simulink model "Gradient_Descent_Sleep_Line_Search"  (R2015a)
settings: Solver=ode3  StartTime=0.0  StopTime=350  FixedStep=0.01  MaxStep=0.01  RelTol=1e-3
values from neighbouring files (symbols this model uses):
  H0 = interp1q(Periodic_Solution(:,1),Periodic_Solution(:,4),time_shift(n))    [Gradient_Descent_Controllable_Sleeping.m]
  Periodic_Solution = Periodic_Solution(Initial_Time*100+1:end,:)    [Gradient_Descent_Controllable_Sleeping.m]    (also in Periodic_Solution_JFK_u_1000lux.mat = [0 0.00999999999999 0.02 0.03 0.04 0.05 0.0599999999999 0.06)
  Sleep0 = 0    [Gradient_Descent_Controllable_Sleeping.m]
  Sleep_update = Sleep    [Gradient_Descent_Controllable_Sleeping.m]
  tol = 0.01    [Gradient_Descent_Controllable_Sleeping.m]
  u_update = u    [Gradient_Descent_Controllable_Sleeping.m]
  x0 = interp1q(Periodic_Solution(:,1),Periodic_Solution(:,2),time_shift(n))    [Gradient_Descent_Controllable_Sleeping.m]
  xc0 = interp1q(Periodic_Solution(:,1),Periodic_Solution(:,3),time_shift(n))    [Gradient_Descent_Controllable_Sleeping.m]
settings Model: Creator=wangf7  LastModifiedBy=Jiawei Yin
settings OptimizationCC: ExpressionDepthLimit=2147483647
settings DebuggingCC: AlgebraicLoopMsg=none  ArtificialAlgebraicLoopMsg=none  UnderspecifiedInitializationDetection=Classic  MergeDetectMultiDrivingBlocksExec=none  SolverPrmCheckMsg=warning  StateNameClashWarn=warning

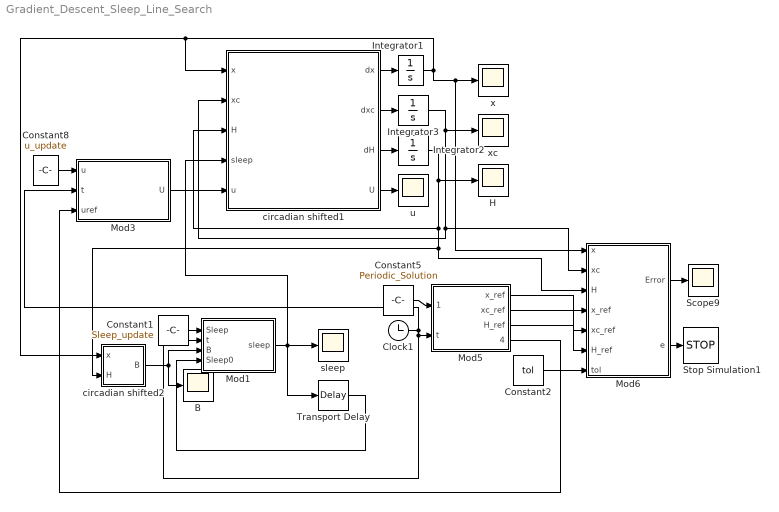
== system Gradient_Descent_Sleep_Line_Search ==
  B : Scope
      settings: TimeRange=auto  MaxDataPoints=5000000000  SaveName=B_plus  YMin=0.1808  YMax=0.82676  SampleTime=-1  DataFormat=Array
  Clock1 : Clock
  Constant1 : Constant  Value=Sleep_update
  Constant2 : Constant  Value=tol
  Constant5 : Constant  Value=Periodic_Solution
  Constant8 : Constant  Value=u_update
  H : Scope
      settings: TimeRange=auto  MaxDataPoints=5000000000  SaveName=H_plus  YMin=0.55428  YMax=0.67222  SampleTime=-1  DataFormat=Array
  Integrator1 : Integrator  InitialCondition=x0
  Integrator2 : Integrator  InitialCondition=H0
  Integrator3 : Integrator  InitialCondition=xc0
  Mod1 : MATLAB Function  TreatAsAtomicUnit=on
      settings: PermitHierarchicalResolution=ParametersOnly
  Mod3 : MATLAB Function  TreatAsAtomicUnit=on
      settings: PermitHierarchicalResolution=ParametersOnly
  Mod5 : MATLAB Function  TreatAsAtomicUnit=on
      settings: PermitHierarchicalResolution=ParametersOnly
  Mod6 : MATLAB Function  TreatAsAtomicUnit=on
      settings: PermitHierarchicalResolution=ParametersOnly
  Scope9 : Scope
      settings: TimeRange=auto  MaxDataPoints=5000000000  SaveName=Error_plus  YMin=-0.4029  YMax=6.32555  SampleTime=-1  DataFormat=Array
  Stop Simulation1 : Stop
  Transport Delay : TransportDelay  DelayTime=.01  InitialOutput=Sleep0
  circadian shifted1 : MATLAB Function  TreatAsAtomicUnit=on
      settings: PermitHierarchicalResolution=ParametersOnly
  circadian shifted2 : MATLAB Function  TreatAsAtomicUnit=on
      settings: PermitHierarchicalResolution=ParametersOnly
  sleep : Scope
      settings: TimeRange=auto  MaxDataPoints=5000000000  SaveName=sleep_plus  YMin=-0.125  YMax=1.125  SampleTime=-1  DataFormat=Array
  u : Scope
      settings: TimeRange=auto  MaxDataPoints=5000000000  SaveName=u_plus  YMin=0.55428  YMax=0.67222  SampleTime=-1  DataFormat=Array
  x : Scope
      settings: TimeRange=auto  MaxDataPoints=5000000000  SaveName=x_plus  YMin=-1.43661  YMax=1.34945  SampleTime=-1  DataFormat=Array
  xc : Scope
      settings: TimeRange=auto  MaxDataPoints=5000000000  SaveName=xc_plus  YMin=0.55428  YMax=0.67222  SampleTime=-1  DataFormat=Array
  wires:
  circadian shifted1/1(dx) -> Integrator1/1
  circadian shifted1/2(dxc) -> Integrator3/1
  Integrator1/1 -> x/1, Mod6/1(x), circadian shifted1/1(x), circadian shifted2/1(x)
  Integrator3/1 -> circadian shifted1/2(xc), Mod6/2(xc), xc/1
  Constant5/1 -> Mod5/1(Periodic_Solution)
  Mod6/2(e) -> Stop Simulation1/1
  Mod6/1(Error) -> Scope9/1
  Mod5/3(H_ref) -> Mod6/6(H_ref)
  Constant2/1 -> Mod6/7(tol)
  Constant1/1 -> Mod1/1(Sleep)
  Clock1/1 -> Mod1/2(t), Mod5/2(t), Mod3/2(t)
  Mod1/1(sleep) -> circadian shifted1/4(sleep), Transport Delay/1, sleep/1
  circadian shifted2/1(B) -> Mod1/3(B), B/1
  Transport Delay/1 -> Mod1/4(Sleep0)
  circadian shifted1/3(dH) -> Integrator2/1
  Integrator2/1 -> Mod6/3(H), circadian shifted2/2(H), circadian shifted1/3(H), H/1
  Mod5/1(x_ref) -> Mod6/4(x_ref)
  Mod5/2(xc_ref) -> Mod6/5(xc_ref)
  Constant8/1 -> Mod3/1(u)
  Mod3/1(U) -> circadian shifted1/5(u)
  circadian shifted1/4(U) -> u/1
  Mod5/4(Sleep_ref) -> Mod3/3(uref)

== matlab function Gradient_Descent_Sleep_Line_Search/circadian shifted1 ==
  data: x input; xc input; H input; sleep input; u input; dx output; dxc output; dH output; U output
function [ dx,dxc,dH,U] = fcn(x,xc,H,sleep,u)
%#eml

tr=18.2;
td=4.2;

q = 1/3;
taux = 24.2;
k = 0.55;
mu=0.13;
U=u*(1-sleep);
B = u*(1-0.4*x)*(1-0.4*xc)*(1-sleep);

dx = (pi/12)*(xc + B  + mu*(1/3*x + 4/3*x^3 - 256/105*x^7));
dxc = (pi/12)*(q*B *xc - (24/(taux*0.99729))^2*x - k*B*x);
dH = (1-sleep)*(1-H)/tr-(H*sleep)/td;

== matlab function Gradient_Descent_Sleep_Line_Search/Mod1 ==
  data: Sleep input; sleep output; t input; B input; Sleep0 input
function sleep = fcn(Sleep,t,B,Sleep0)
%#codegen
if t<=Sleep(end,1)
    sleep=interp1q(Sleep(:,1),Sleep(:,2),t);
    if sleep==0 && Sleep0==1
        if B>0.27
            sleep=1;
        end
    elseif sleep==1 && Sleep0==0
        if B<0.67
            sleep=0;
        end
    end
    if B>0.77
        sleep=1;
    elseif B<0.17
        sleep=0;
    end
else
    sleep=Sleep0;
    if B>0.67
        sleep=1;
    elseif B<0.17
        sleep=0;
    end
end

== matlab function Gradient_Descent_Sleep_Line_Search/circadian shifted2 ==
  data: x input; H input; B output
function B = fcn(x,H)
%#eml
B=H-0.1333*x;

== matlab function Gradient_Descent_Sleep_Line_Search/Mod5 ==
  data: Periodic_Solution input; x_ref output; xc_ref output; t input; H_ref output; Sleep_ref output
function [x_ref,xc_ref,H_ref,Sleep_ref] = fcn(Periodic_Solution,t)
%#codegen
x_ref=interp1q(Periodic_Solution(:,1),Periodic_Solution(:,2),t);
xc_ref=interp1q(Periodic_Solution(:,1),Periodic_Solution(:,3),t);
H_ref=interp1q(Periodic_Solution(:,1),Periodic_Solution(:,4),t);
% Sleep_ref=interp1q(Periodic_Solution(:,1),Periodic_Solution(:,6),t);
Sleep_ref=interp1q(Periodic_Solution(:,1),Periodic_Solution(:,5),t);

== matlab function Gradient_Descent_Sleep_Line_Search/Mod6 ==
  data: Error output; x input; xc input; H input; x_ref input; xc_ref input; H_ref input; e output; tol input
function [Error,e] = fcn(x,xc,H,x_ref,xc_ref,H_ref,tol)
%#codegen
Error=(H-H_ref)^2+(x-x_ref)^2+(xc-xc_ref)^2;
e=Error<tol;

== matlab function Gradient_Descent_Sleep_Line_Search/Mod3 ==
  data: u input; U output; t input; uref input
function U  = fcn(u,t,uref)
%#codegen
if t<=u(end,1)
    U=interp1q(u(:,1),u(:,2),t);
else
    U=uref;
end
